simulink model "ackerman_modelo_parte1_neuronal"  (R2023b)
settings: Solver=FixedStepDiscrete  StartTime=0.0  StopTime=50  FixedStep=0.1  RelTol=1e-3
undefined symbols (not defined in the file or in its folder): Angular, Linear
libraries: neural x121, robotlib x15, fuzblock x1, robotcorelib x1
(part 4 of 5)

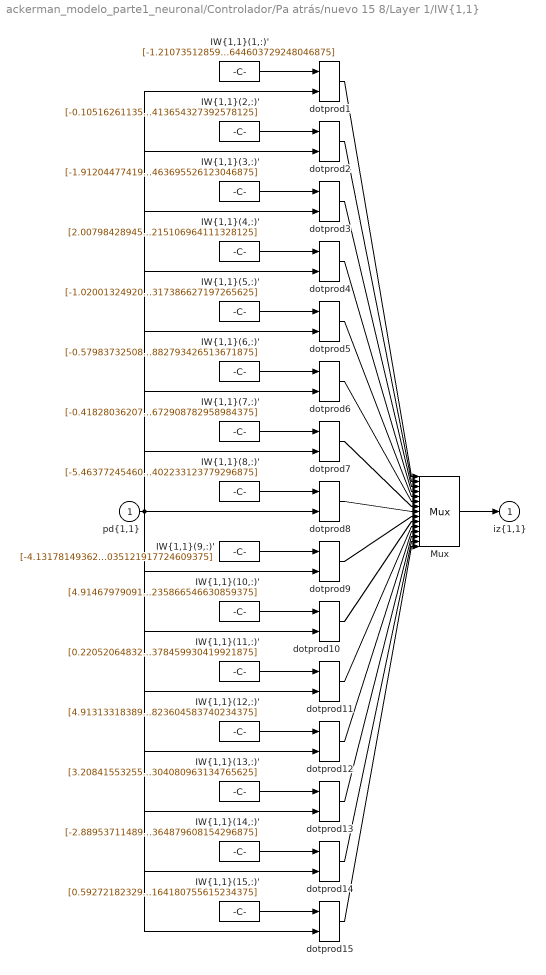
== system ackerman_modelo_parte1_neuronal/Controlador/Pa atrás/nuevo 15 8/Layer 1/IW{1,1} ==
  "pd{1,1}" : Inport  PortDimensions=12  SampleTime=0.1
      mask Display: e = 0.06;c1 = [120 230 180]/255;c2 = ([120 230 180]+0)/(256+128);c3 = ([120 230 180]+128)/(256+128);patch([0 1 1 0],[0 0 1 1],c1);patch([0 1 1 1-e 1-e 0+e],[0 0 1 1-e 0+e 0+e],c2);patch([0 0 1 1-e 0+e 0+e],[0 1 1 1-e 1-e 0+e],c3);plot([0 1 1 0 0],[0 0 1 1 0]);
  "IW{1,1}(1,:)'" : Constant  Value=[-1.2107351285968033227646856175852008163928985595703125;0.0982637498885013116467490590366651304066181182861328125;-0.5153760046711977071964838614803738892078399658203125;4.31122767760680147830498754046857357025146484375;3.85293074004639368723701409180648624897003173828125;-0.210691315343805418702771703465259633958339691162109375;2.04507854540902034301552703254856169223785400390625;-0.9143036407233731122090603093965910375118255615234375;-0.0603308152257395757800395585945807397365570068359375;-1.4964433902647422680587396826012991368770599365234375;0.70598829467948298610480151182855479419231414794921875;-3.888548718957604677370909485034644603729248046875]
      mask Display: e = 0.06;c1 = [120 150 230]/255;c2 = ([120 150 230]+0)/383;c3 = ([120 150 230]+128)/383;patch([0 1 1 0],[0 0 1 1],c1);patch([0 1 1 1-e 1-e 0+e],[0 0 1 1-e 0+e 0+e],c2);patch([0 0 1 1-e 0+e 0+e],[0 1 1 1-e 1-e 0+e],c3);plot([0 1 1 0 0],[0 0 1 1 0]);disp('Weights');
  "IW{1,1}(10,:)'" : Constant  Value=[4.91467979091452367157444314216263592243194580078125;4.34626894631366322840904103941284120082855224609375;2.404366244111241446290705425781197845935821533203125;-6.8842796230847458360813106992281973361968994140625;2.139509471626407588473739451728761196136474609375;3.83863946131409239370668728952296078205108642578125;-3.39886262811612649414882980636321008205413818359375;-3.524387185952170487013290767208673059940338134765625;3.065775570742113931288486128323711454868316650390625;1.4407812730284497160226919731940142810344696044921875;0.08745738485305031006955545080927549861371517181396484375;0.85647591674319922816493999562226235866546630859375]
      mask Display: e = 0.06;c1 = [120 150 230]/255;c2 = ([120 150 230]+0)/383;c3 = ([120 150 230]+128)/383;patch([0 1 1 0],[0 0 1 1],c1);patch([0 1 1 1-e 1-e 0+e],[0 0 1 1-e 0+e 0+e],c2);patch([0 0 1 1-e 0+e 0+e],[0 1 1 1-e 1-e 0+e],c3);plot([0 1 1 0 0],[0 0 1 1 0]);disp('Weights');
  "IW{1,1}(11,:)'" : Constant  Value=[0.2205206483206818557363249055924825370311737060546875;1.8123150518481307980067640528432093560695648193359375;0.7869633308428676254919764687656424939632415771484375;2.18414976750363099000651345704682171344757080078125;-3.05959657538790086306335069821216166019439697265625;2.11925190216866621284452776308171451091766357421875;-0.222273935716689352570796245345263741910457611083984375;-0.5932835817560018210059524790267460048198699951171875;0.9675585951395404560315682829241268336772918701171875;-2.879213642821424112838712972006760537624359130859375;-0.936850701180139910917432644055224955081939697265625;-0.99529495461161854308329566265456378459930419921875]
      mask Display: e = 0.06;c1 = [120 150 230]/255;c2 = ([120 150 230]+0)/383;c3 = ([120 150 230]+128)/383;patch([0 1 1 0],[0 0 1 1],c1);patch([0 1 1 1-e 1-e 0+e],[0 0 1 1-e 0+e 0+e],c2);patch([0 0 1 1-e 0+e 0+e],[0 1 1 1-e 1-e 0+e],c3);plot([0 1 1 0 0],[0 0 1 1 0]);disp('Weights');
  "IW{1,1}(12,:)'" : Constant  Value=[4.91313318389939457375703568686731159687042236328125;-0.2228704482321312851933470255971769802272319793701171875;1.48781041301915362140562137938104569911956787109375;2.11504413384102374351414255215786397457122802734375;-5.6137042363568081526636888156644999980926513671875;-0.868753373670580142373864873661659657955169677734375;3.59322897737675095442000383627600967884063720703125;0.54487347859706491970399611091124825179576873779296875;6.037217866595415927122303401120007038116455078125;-3.333595774710569781262847754987888038158416748046875;2.317143802646336236961133181466720998287200927734375;0.08013759538293162287825310841071768663823604583740234375]
      mask Display: e = 0.06;c1 = [120 150 230]/255;c2 = ([120 150 230]+0)/383;c3 = ([120 150 230]+128)/383;patch([0 1 1 0],[0 0 1 1],c1);patch([0 1 1 1-e 1-e 0+e],[0 0 1 1-e 0+e 0+e],c2);patch([0 0 1 1-e 0+e 0+e],[0 1 1 1-e 1-e 0+e],c3);plot([0 1 1 0 0],[0 0 1 1 0]);disp('Weights');
  "IW{1,1}(13,:)'" : Constant  Value=[3.2084155325522534241144967381842434406280517578125;4.08655173187908982157523496425710618495941162109375;-0.74005314094400909130655463741277344524860382080078125;-1.4115221687797758765015032622613944113254547119140625;-4.52962761692046544936829377547837793827056884765625;-3.25902700111771448376885018660686910152435302734375;-2.27197968931137861403612987487576901912689208984375;-1.6041119526664726624431978052598424255847930908203125;1.7664155094637392640066764215589500963687896728515625;-1.9371624002321834456807891911012120544910430908203125;4.80163975118690444787716842256486415863037109375;2.7784505359702027504908983246423304080963134765625]
      mask Display: e = 0.06;c1 = [120 150 230]/255;c2 = ([120 150 230]+0)/383;c3 = ([120 150 230]+128)/383;patch([0 1 1 0],[0 0 1 1],c1);patch([0 1 1 1-e 1-e 0+e],[0 0 1 1-e 0+e 0+e],c2);patch([0 0 1 1-e 0+e 0+e],[0 1 1 1-e 1-e 0+e],c3);plot([0 1 1 0 0],[0 0 1 1 0]);disp('Weights');
  "IW{1,1}(14,:)'" : Constant  Value=[-2.889537114898974135002163166063837707042694091796875;-1.048370824648822807745318641536869108676910400390625;-0.51568992051216977490213366763782687485218048095703125;0.0980394159708294632427083570291870273649692535400390625;0.1474327544041719451062277812525280751287937164306640625;-1.9644717917155867237255506552173756062984466552734375;-3.141171661324176245244643723708577454090118408203125;-2.1627338507038214032718315138481557369232177734375;-2.283212601949863529426920649711973965167999267578125;0.2879837913213993960681591488537378609180450439453125;-1.6861613409542035579846697146422229707241058349609375;-0.90119074943709509550870961902546696364879608154296875]
      mask Display: e = 0.06;c1 = [120 150 230]/255;c2 = ([120 150 230]+0)/383;c3 = ([120 150 230]+128)/383;patch([0 1 1 0],[0 0 1 1],c1);patch([0 1 1 1-e 1-e 0+e],[0 0 1 1-e 0+e 0+e],c2);patch([0 0 1 1-e 0+e 0+e],[0 1 1 1-e 1-e 0+e],c3);plot([0 1 1 0 0],[0 0 1 1 0]);disp('Weights');
  "IW{1,1}(15,:)'" : Constant  Value=[0.5927218232989857060744043337763287127017974853515625;6.05095360760331058003202997497282922267913818359375;5.70459075526748815576638662605546414852142333984375;1.0913370531196016077757349194143898785114288330078125;-6.16238780094926763553075943491421639919281005859375;3.14740655635683896917953461525030434131622314453125;1.6970071893540310536963033882784657180309295654296875;-1.74537787608898664615253437659703195095062255859375;0.214836119473990672101848531383438967168331146240234375;4.3552918607225450386977172456681728363037109375;3.99437144434348123667177787865512073040008544921875;3.0011419277898792046244125231169164180755615234375]
      mask Display: e = 0.06;c1 = [120 150 230]/255;c2 = ([120 150 230]+0)/383;c3 = ([120 150 230]+128)/383;patch([0 1 1 0],[0 0 1 1],c1);patch([0 1 1 1-e 1-e 0+e],[0 0 1 1-e 0+e 0+e],c2);patch([0 0 1 1-e 0+e 0+e],[0 1 1 1-e 1-e 0+e],c3);plot([0 1 1 0 0],[0 0 1 1 0]);disp('Weights');
  "IW{1,1}(2,:)'" : Constant  Value=[-0.1051626113599678780108348519206629134714603424072265625;-5.083606135239737255915315472520887851715087890625;2.00321524443686005412246231571771204471588134765625;0.86672090627960673980823003148543648421764373779296875;2.228908768658861117017977448995225131511688232421875;-0.80080397013559767582790982487495057284832000732421875;0.49174544290695099135746204410679638385772705078125;3.6915718186289350200013359426520764827728271484375;-1.19836535767401830554490516078658401966094970703125;-1.706882284913678216042853819089941680431365966796875;-0.822687260484902704860132871544919908046722412109375;0.70350327650940791546219088559155352413654327392578125]
      mask Display: e = 0.06;c1 = [120 150 230]/255;c2 = ([120 150 230]+0)/383;c3 = ([120 150 230]+128)/383;patch([0 1 1 0],[0 0 1 1],c1);patch([0 1 1 1-e 1-e 0+e],[0 0 1 1-e 0+e 0+e],c2);patch([0 0 1 1-e 0+e 0+e],[0 1 1 1-e 1-e 0+e],c3);plot([0 1 1 0 0],[0 0 1 1 0]);disp('Weights');
  "IW{1,1}(3,:)'" : Constant  Value=[-1.9120447741941515307217969166231341660022735595703125;-0.456778138788140608550492061112890951335430145263671875;0.61407563958637301215759407568839378654956817626953125;-0.59789275549836140566384301564539782702922821044921875;-3.52278262027996991179179531172849237918853759765625;2.111624613374857961645147952367551624774932861328125;-3.9493715623728125052593895816244184970855712890625;1.10848913770916279730727183050476014614105224609375;4.96544220863601548643373462255112826824188232421875;-2.521311409694160676764340678346343338489532470703125;-4.376974089342962059845376643352210521697998046875;2.135437127611392593706796105834655463695526123046875]
      mask Display: e = 0.06;c1 = [120 150 230]/255;c2 = ([120 150 230]+0)/383;c3 = ([120 150 230]+128)/383;patch([0 1 1 0],[0 0 1 1],c1);patch([0 1 1 1-e 1-e 0+e],[0 0 1 1-e 0+e 0+e],c2);patch([0 0 1 1-e 0+e 0+e],[0 1 1 1-e 1-e 0+e],c3);plot([0 1 1 0 0],[0 0 1 1 0]);disp('Weights');
  "IW{1,1}(4,:)'" : Constant  Value=[2.0079842894568162847690473427064716815948486328125;0.77019648946443652892668296772171743214130401611328125;3.1709271112167289885519494418986141681671142578125;-1.2126101810723934892877196034532971680164337158203125;-4.377744816317044040943073923699557781219482421875;3.143535997099470069571225394611246883869171142578125;6.37228009121002259007582324557006359100341796875;5.3420881020253947468745536752976477146148681640625;-0.1580693080755513069135531623032875359058380126953125;0.916039178029972145367310076835565268993377685546875;4.446636562875664111516016419045627117156982421875;0.85009214377447250843289339172770269215106964111328125]
      mask Display: e = 0.06;c1 = [120 150 230]/255;c2 = ([120 150 230]+0)/383;c3 = ([120 150 230]+128)/383;patch([0 1 1 0],[0 0 1 1],c1);patch([0 1 1 1-e 1-e 0+e],[0 0 1 1-e 0+e 0+e],c2);patch([0 0 1 1-e 0+e 0+e],[0 1 1 1-e 1-e 0+e],c3);plot([0 1 1 0 0],[0 0 1 1 0]);disp('Weights');
  "IW{1,1}(5,:)'" : Constant  Value=[-1.0200132492011257934194645713432691991329193115234375;2.115587292969216104410179468686692416667938232421875;0.058765464456745297727735533044324256479740142822265625;-0.9369911708232419034203530827653594315052032470703125;-0.8617614761682770296857825087499804794788360595703125;-2.436977052131390042433167764102108776569366455078125;-1.9178939983275438141419044768554158508777618408203125;-3.657381782514789403393251632223837077617645263671875;0.0727938413210702239819482883831369690597057342529296875;5.3628189763214226815080110100097954273223876953125;-1.9620170434064068132329339277930557727813720703125;0.60265908988629723896934820004389621317386627197265625]
      mask Display: e = 0.06;c1 = [120 150 230]/255;c2 = ([120 150 230]+0)/383;c3 = ([120 150 230]+128)/383;patch([0 1 1 0],[0 0 1 1],c1);patch([0 1 1 1-e 1-e 0+e],[0 0 1 1-e 0+e 0+e],c2);patch([0 0 1 1-e 0+e 0+e],[0 1 1 1-e 1-e 0+e],c3);plot([0 1 1 0 0],[0 0 1 1 0]);disp('Weights');
  "IW{1,1}(6,:)'" : Constant  Value=[-0.5798373250875332729492583894170820713043212890625;3.49037173488871221849194625974632799625396728515625;2.69385366427376293785300731542520225048065185546875;4.99342327369683491866680924431420862674713134765625;1.3203490130336168473235147757804952561855316162109375;0.68025931851506127312489979885867796838283538818359375;5.04882126855442958657249619136564433574676513671875;-2.352048108762541556160385880502872169017791748046875;-5.6367484957371818410365449381060898303985595703125;1.343725558897456817675220008823089301586151123046875;-1.028824242655661524992183331050910055637359619140625;-3.479813826287624589639335681567899882793426513671875]
      mask Display: e = 0.06;c1 = [120 150 230]/255;c2 = ([120 150 230]+0)/383;c3 = ([120 150 230]+128)/383;patch([0 1 1 0],[0 0 1 1],c1);patch([0 1 1 1-e 1-e 0+e],[0 0 1 1-e 0+e 0+e],c2);patch([0 0 1 1-e 0+e 0+e],[0 1 1 1-e 1-e 0+e],c3);plot([0 1 1 0 0],[0 0 1 1 0]);disp('Weights');
  "IW{1,1}(7,:)'" : Constant  Value=[-0.41828036207490260078856181280571036040782928466796875;-3.207646797774704960914959883666597306728363037109375;1.118927025324791824090198133490048348903656005859375;-0.85184466732525565557665458982228301465511322021484375;-0.507459282776808517922972896485589444637298583984375;-0.00546286069858389726483505199894352699629962444305419921875;-1.0917087277428538794055157268303446471691131591796875;1.6598742597553126643106224946677684783935546875;-2.34331138125278659600780883920378983020782470703125;-2.455131769084918591516952801612205803394317626953125;-1.2118189054765855505735316910431720316410064697265625;-2.27290972117965761611912967055104672908782958984375]
      mask Display: e = 0.06;c1 = [120 150 230]/255;c2 = ([120 150 230]+0)/383;c3 = ([120 150 230]+128)/383;patch([0 1 1 0],[0 0 1 1],c1);patch([0 1 1 1-e 1-e 0+e],[0 0 1 1-e 0+e 0+e],c2);patch([0 0 1 1-e 0+e 0+e],[0 1 1 1-e 1-e 0+e],c3);plot([0 1 1 0 0],[0 0 1 1 0]);disp('Weights');
  "IW{1,1}(8,:)'" : Constant  Value=[-5.46377245460134730592471896670758724212646484375;4.77850376478235272514893949846737086772918701171875;-3.063882030696078562215234342147596180438995361328125;1.7026186023976028760529288774705491960048675537109375;0.057268640450032416711056981739602633751928806304931640625;-3.043911938405681194552698798361234366893768310546875;-2.087085973080445189253850912791676819324493408203125;-0.6478883460483615408520563505589962005615234375;-1.6495490128681875585670013606431894004344940185546875;3.76449083714243304399360567913390696048736572265625;-2.061732774841388948772191724856384098529815673828125;0.440287490512660528718669183945166878402233123779296875]
      mask Display: e = 0.06;c1 = [120 150 230]/255;c2 = ([120 150 230]+0)/383;c3 = ([120 150 230]+128)/383;patch([0 1 1 0],[0 0 1 1],c1);patch([0 1 1 1-e 1-e 0+e],[0 0 1 1-e 0+e 0+e],c2);patch([0 0 1 1-e 0+e 0+e],[0 1 1 1-e 1-e 0+e],c3);plot([0 1 1 0 0],[0 0 1 1 0]);disp('Weights');
  "IW{1,1}(9,:)'" : Constant  Value=[-4.1317814936234071865328587591648101806640625;-0.54267309292749998927973820173065178096294403076171875;3.248198500675273603377490871935151517391204833984375;2.314857084656230856722913813428021967411041259765625;1.8523167152062758322728086568531580269336700439453125;1.9029771433222639753779503735131584107875823974609375;3.357464691081492258462048994260840117931365966796875;-1.8211175913287707128773718068259768187999725341796875;2.871623886888575949427604427910409867763519287109375;3.300857412961221815095314013888128101825714111328125;-8.9937746890157530543774555553682148456573486328125;2.118140016172025408280887859291397035121917724609375]
      mask Display: e = 0.06;c1 = [120 150 230]/255;c2 = ([120 150 230]+0)/383;c3 = ([120 150 230]+128)/383;patch([0 1 1 0],[0 0 1 1],c1);patch([0 1 1 1-e 1-e 0+e],[0 0 1 1-e 0+e 0+e],c2);patch([0 0 1 1-e 0+e 0+e],[0 1 1 1-e 1-e 0+e],c3);plot([0 1 1 0 0],[0 0 1 1 0]);disp('Weights');
  Mux : Mux  Inputs=15
      mask Display: e = 0.06;c1 = [120 150 230]/255;c2 = ([120 150 230]+0)/383;c3 = ([120 150 230]+128)/383;patch([0 1 1 0],[0 0 1 1],c1);patch([0 1 1 1-e 1-e 0+e],[0 0 1 1-e 0+e 0+e],c2);patch([0 0 1 1-e 0+e 0+e],[0 1 1 1-e 1-e 0+e],c3);plot([0 1 1 0 0],[0 0 1 1 0]);disp('Mux');
  dotprod{1..15} (15 alike) : neural/Weight Functions/dotprod
  "iz{1,1}" : Outport
      mask Display: e = 0.06;c1 = [120 230 180]/255;c2 = ([120 230 180]+0)/(256+128);c3 = ([120 230 180]+128)/(256+128);patch([0 1 1 0],[0 0 1 1],c1);patch([0 1 1 1-e 1-e 0+e],[0 0 1 1-e 0+e 0+e],c2);patch([0 0 1 1-e 0+e 0+e],[0 1 1 1-e 1-e 0+e],c3);plot([0 1 1 0 0],[0 0 1 1 0]);
  wires:
  Mux/1 -> "iz{1,1}"/1
  dotprod15/1 -> Mux/15
  "IW{1,1}(15,:)'"/1 -> dotprod15/1
  dotprod14/1 -> Mux/14
  "IW{1,1}(14,:)'"/1 -> dotprod14/1
  dotprod13/1 -> Mux/13
  "IW{1,1}(13,:)'"/1 -> dotprod13/1
  dotprod12/1 -> Mux/12
  "IW{1,1}(12,:)'"/1 -> dotprod12/1
  dotprod11/1 -> Mux/11
  "IW{1,1}(11,:)'"/1 -> dotprod11/1
  dotprod10/1 -> Mux/10
  "IW{1,1}(10,:)'"/1 -> dotprod10/1
  dotprod9/1 -> Mux/9
  "IW{1,1}(9,:)'"/1 -> dotprod9/1
  dotprod8/1 -> Mux/8
  "IW{1,1}(8,:)'"/1 -> dotprod8/1
  dotprod7/1 -> Mux/7
  "IW{1,1}(7,:)'"/1 -> dotprod7/1
  dotprod6/1 -> Mux/6
  "IW{1,1}(6,:)'"/1 -> dotprod6/1
  dotprod5/1 -> Mux/5
  "IW{1,1}(5,:)'"/1 -> dotprod5/1
  dotprod4/1 -> Mux/4
  "IW{1,1}(4,:)'"/1 -> dotprod4/1
  dotprod3/1 -> Mux/3
  "IW{1,1}(3,:)'"/1 -> dotprod3/1
  dotprod2/1 -> Mux/2
  "IW{1,1}(2,:)'"/1 -> dotprod2/1
  dotprod1/1 -> Mux/1
  "pd{1,1}"/1 -> dotprod15/2, dotprod14/2, dotprod13/2, dotprod12/2, dotprod11/2, dotprod10/2, dotprod9/2, dotprod8/2, dotprod7/2, dotprod6/2, dotprod5/2, dotprod4/2, dotprod3/2, dotprod2/2, dotprod1/2
  "IW{1,1}(1,:)'"/1 -> dotprod1/1

== system ackerman_modelo_parte1_neuronal/Controlador/Pa atrás/nuevo 15 8/Layer 2/Delays 1 ==
  "p{2}" : Inport  PortDimensions=15  SampleTime=0.1
      mask Display: e = 0.06;c1 = [120 230 180]/255;c2 = ([120 230 180]+0)/(256+128);c3 = ([120 230 180]+128)/(256+128);patch([0 1 1 0],[0 0 1 1],c1);patch([0 1 1 1-e 1-e 0+e],[0 0 1 1-e 0+e 0+e],c2);patch([0 0 1 1-e 0+e 0+e],[0 1 1 1-e 1-e 0+e],c3);plot([0 1 1 0 0],[0 0 1 1 0]);
  mux : Mux  Inputs=1
      mask Display: e = 0.06;c1 = [120 150 230]/255;c2 = ([120 150 230]+0)/383;c3 = ([120 150 230]+128)/383;patch([0 1 1 0],[0 0 1 1],c1);patch([0 1 1 1-e 1-e 0+e],[0 0 1 1-e 0+e 0+e],c2);patch([0 0 1 1-e 0+e 0+e],[0 1 1 1-e 1-e 0+e],c3);plot([0 1 1 0 0],[0 0 1 1 0]);disp('Mux')
  "pd{2,1}" : Outport
      mask Display: e = 0.06;c1 = [120 230 180]/255;c2 = ([120 230 180]+0)/(256+128);c3 = ([120 230 180]+128)/(256+128);patch([0 1 1 0],[0 0 1 1],c1);patch([0 1 1 1-e 1-e 0+e],[0 0 1 1-e 0+e 0+e],c2);patch([0 0 1 1-e 0+e 0+e],[0 1 1 1-e 1-e 0+e],c3);plot([0 1 1 0 0],[0 0 1 1 0]);
  wires:
  mux/1 -> "pd{2,1}"/1
  "p{2}"/1 -> mux/1

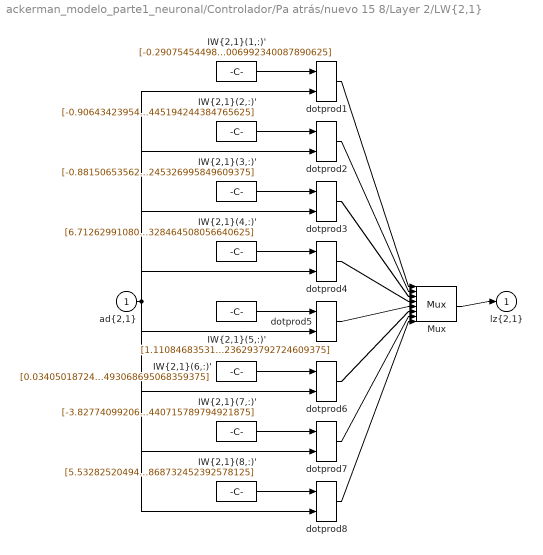
== system ackerman_modelo_parte1_neuronal/Controlador/Pa atrás/nuevo 15 8/Layer 2/LW{2,1} ==
  "ad{2,1}" : Inport  PortDimensions=15  SampleTime=0.1
      mask Display: e = 0.06;c1 = [120 230 180]/255;c2 = ([120 230 180]+0)/(256+128);c3 = ([120 230 180]+128)/(256+128);patch([0 1 1 0],[0 0 1 1],c1);patch([0 1 1 1-e 1-e 0+e],[0 0 1 1-e 0+e 0+e],c2);patch([0 0 1 1-e 0+e 0+e],[0 1 1 1-e 1-e 0+e],c3);plot([0 1 1 0 0],[0 0 1 1 0]);
  "IW{2,1}(1,:)'" : Constant  Value=[-0.29075454498602126829354119763593189418315887451171875;-0.98812314853822424964846504735760390758514404296875;0.711716360142102377750461528194136917591094970703125;0.90234703837315477503722149776876904070377349853515625;0.8126684356467970271609146948321722447872161865234375;-1.74164913561031564626091494574211537837982177734375;2.376338350655095243979531005606986582279205322265625;-0.92238662868760024071690395430778153240680694580078125;0.050248126972542821178091543288246612064540386199951171875;0.697568123453101041064883247599937021732330322265625;0.24326358760592459162808154360391199588775634765625;1.4125306528485872537004297555540688335895538330078125;0.539762979340757897972480350290425121784210205078125;2.241164585342918513788390555419027805328369140625;-0.96705426576078290512583635063492693006992340087890625]
      mask Display: e = 0.06;c1 = [120 150 230]/255;c2 = ([120 150 230]+0)/383;c3 = ([120 150 230]+128)/383;patch([0 1 1 0],[0 0 1 1],c1);patch([0 1 1 1-e 1-e 0+e],[0 0 1 1-e 0+e 0+e],c2);patch([0 0 1 1-e 0+e 0+e],[0 1 1 1-e 1-e 0+e],c3);plot([0 1 1 0 0],[0 0 1 1 0]);disp('weights');
  "IW{2,1}(2,:)'" : Constant  Value=[-0.906434239547387665680844293092377483844757080078125;-0.97475679697394335132543119470938108861446380615234375;-0.246538118535185868385184448925429023802280426025390625;-0.32752283539170956583319593846681527793407440185546875;-0.4956324478575202530095111796981655061244964599609375;-0.9529361012520130014280539398896507918834686279296875;0.8396212024492586412094397019245661795139312744140625;0.40149777369720640596284511047997511923313140869140625;4.930764217762515499998698942363262176513671875;0.19805403441289104460309999922174029052257537841796875;-0.38628534525447222325311713575501926243305206298828125;-0.2381274587910517659405940094075049273669719696044921875;-1.0404188470728821247490714085870422422885894775390625;-1.1803335311705318577679690861259587109088897705078125;-0.260692367339245001378600363750592805445194244384765625]
      mask Display: e = 0.06;c1 = [120 150 230]/255;c2 = ([120 150 230]+0)/383;c3 = ([120 150 230]+128)/383;patch([0 1 1 0],[0 0 1 1],c1);patch([0 1 1 1-e 1-e 0+e],[0 0 1 1-e 0+e 0+e],c2);patch([0 0 1 1-e 0+e 0+e],[0 1 1 1-e 1-e 0+e],c3);plot([0 1 1 0 0],[0 0 1 1 0]);disp('weights');
  "IW{2,1}(3,:)'" : Constant  Value=[-0.8815065356279401243000393151305615901947021484375;-2.172966928915788020759691789862699806690216064453125;0.6199742002492651948841739795170724391937255859375;1.59509701476742460357627351186238229274749755859375;-0.49622943112802442300335314939729869365692138671875;-0.52170933231938387830695091906818561255931854248046875;2.065467985535988315604072340647689998149871826171875;0.82253371757050819379486483740038238465785980224609375;-1.2643496444477679840900918861734680831432342529296875;-1.96010366548021419674796561594121158123016357421875;-5.18390017704719152646930524497292935848236083984375;1.799562773148688510360670989030040800571441650390625;-0.6347599582949925434149918146431446075439453125;3.202342757938753781132845688262023031711578369140625;2.29683725330840271539045716053806245326995849609375]
      mask Display: e = 0.06;c1 = [120 150 230]/255;c2 = ([120 150 230]+0)/383;c3 = ([120 150 230]+128)/383;patch([0 1 1 0],[0 0 1 1],c1);patch([0 1 1 1-e 1-e 0+e],[0 0 1 1-e 0+e 0+e],c2);patch([0 0 1 1-e 0+e 0+e],[0 1 1 1-e 1-e 0+e],c3);plot([0 1 1 0 0],[0 0 1 1 0]);disp('weights');
  "IW{2,1}(4,:)'" : Constant  Value=[6.712629910804526645051737432368099689483642578125;2.685481115080815772699907029164023697376251220703125;-5.22242244096624830262953764759004116058349609375;-4.64646258408361489955495926551520824432373046875;-7.8937720699343909558365339762531220912933349609375;-1.489316993595450444587413585395552217960357666015625;-0.0012315191105431166906925000148476101458072662353515625;-2.45356904701287703574053011834621429443359375;-4.3445683416797660214569987147115170955657958984375;9.4684540456393051499617286026477813720703125;-0.0495316660597107105701297768973745405673980712890625;7.388094109720238833460825844667851924896240234375;-7.59068304960720841023658067570067942142486572265625;-5.03963279409498188243787808460183441638946533203125;-5.151307660039666558304816135205328464508056640625]
      mask Display: e = 0.06;c1 = [120 150 230]/255;c2 = ([120 150 230]+0)/383;c3 = ([120 150 230]+128)/383;patch([0 1 1 0],[0 0 1 1],c1);patch([0 1 1 1-e 1-e 0+e],[0 0 1 1-e 0+e 0+e],c2);patch([0 0 1 1-e 0+e 0+e],[0 1 1 1-e 1-e 0+e],c3);plot([0 1 1 0 0],[0 0 1 1 0]);disp('weights');
  "IW{2,1}(5,:)'" : Constant  Value=[1.11084683531153505242627943516708910465240478515625;3.10043446301388403441023911000229418277740478515625;-1.0134746863376646874854714042157866060733795166015625;-1.770345289966909430035002515069209039211273193359375;-0.2142097084749770286027370502779376693069934844970703125;0.458936962485257449184672395858797244727611541748046875;-1.4054444424488057308053612359799444675445556640625;-0.68180700087420464949872211946058087050914764404296875;2.66641420630732550733910102280788123607635498046875;2.97762361888042192958891973830759525299072265625;3.51435835506861860011440512607805430889129638671875;-1.8125822622395599825750878153485246002674102783203125;1.022824479711518907976142145344056189060211181640625;-3.957830076097492710829328643740154802799224853515625;-2.850774159259832796209366279072128236293792724609375]
      mask Display: e = 0.06;c1 = [120 150 230]/255;c2 = ([120 150 230]+0)/383;c3 = ([120 150 230]+128)/383;patch([0 1 1 0],[0 0 1 1],c1);patch([0 1 1 1-e 1-e 0+e],[0 0 1 1-e 0+e 0+e],c2);patch([0 0 1 1-e 0+e 0+e],[0 1 1 1-e 1-e 0+e],c3);plot([0 1 1 0 0],[0 0 1 1 0]);disp('weights');
  "IW{2,1}(6,:)'" : Constant  Value=[0.0340501872422650786464970451561384834349155426025390625;-1.2045003328454597646413049005786888301372528076171875;-1.0884166133174826285312519758008420467376708984375;0.3230741253505637899934299639426171779632568359375;-0.69639101967878414001233977614901959896087646484375;-3.089062141086427626390786826959811151027679443359375;1.4201511556334318608918465542956255376338958740234375;-4.16687048502832357854686051723547279834747314453125;2.133040159648561751026818456011824309825897216796875;0.82352929019639253827023139820084907114505767822265625;-0.70289762206718087167445219165529124438762664794921875;-1.85767819933412869914945986238308250904083251953125;-7.98033056572949117679627306642942130565643310546875;-0.100894081643059629893599549177451990544795989990234375;-0.2212247530592440225571948531069210730493068695068359375]
      mask Display: e = 0.06;c1 = [120 150 230]/255;c2 = ([120 150 230]+0)/383;c3 = ([120 150 230]+128)/383;patch([0 1 1 0],[0 0 1 1],c1);patch([0 1 1 1-e 1-e 0+e],[0 0 1 1-e 0+e 0+e],c2);patch([0 0 1 1-e 0+e 0+e],[0 1 1 1-e 1-e 0+e],c3);plot([0 1 1 0 0],[0 0 1 1 0]);disp('weights');
  "IW{2,1}(7,:)'" : Constant  Value=[-3.827740992069419423415865821880288422107696533203125;-1.803984388809799721542503903037868440151214599609375;-1.822978187467001465194016418536193668842315673828125;5.97278661820225931222694271127693355083465576171875;-0.46747572108686774594588086984003894031047821044921875;2.19118725790278912057829074910841882228851318359375;5.15945985602581647100350892287679016590118408203125;-0.108402320187160394748815406273934058845043182373046875;4.174033651074037010175743489526212215423583984375;1.1081929070829825700883475292357616126537322998046875;-2.91075125748298457750706802471540868282318115234375;1.8023160883693958300710846742731519043445587158203125;0.30533085219115052577620872398256324231624603271484375;-5.911244402832952715698411338962614536285400390625;-1.1969564893468322974712236828054301440715789794921875]
      mask Display: e = 0.06;c1 = [120 150 230]/255;c2 = ([120 150 230]+0)/383;c3 = ([120 150 230]+128)/383;patch([0 1 1 0],[0 0 1 1],c1);patch([0 1 1 1-e 1-e 0+e],[0 0 1 1-e 0+e 0+e],c2);patch([0 0 1 1-e 0+e 0+e],[0 1 1 1-e 1-e 0+e],c3);plot([0 1 1 0 0],[0 0 1 1 0]);disp('weights');
  "IW{2,1}(8,:)'" : Constant  Value=[5.53282520494231189189804354100488126277923583984375;-2.37112003554331796095766549115069210529327392578125;4.7693327640777152254258908214978873729705810546875;-11.451800696300239224001416005194187164306640625;0.9340318427855525129643865511752665042877197265625;-0.368663405563989965418869587665540166199207305908203125;0.4524664595962504254345049048424698412418365478515625;-1.7536704038506008007658465430722571909427642822265625;-4.7963403600431373519086264423094689846038818359375;0.0099681725079447114357122927685850299894809722900390625;2.877485348191205272172510376549325883388519287109375;0.81593620475731665209195853094570338726043701171875;4.48453559542245283608963291044346988201141357421875;1.845719256720041556718570063821971416473388671875;3.259645459578770942954406564240343868732452392578125]
      mask Display: e = 0.06;c1 = [120 150 230]/255;c2 = ([120 150 230]+0)/383;c3 = ([120 150 230]+128)/383;patch([0 1 1 0],[0 0 1 1],c1);patch([0 1 1 1-e 1-e 0+e],[0 0 1 1-e 0+e 0+e],c2);patch([0 0 1 1-e 0+e 0+e],[0 1 1 1-e 1-e 0+e],c3);plot([0 1 1 0 0],[0 0 1 1 0]);disp('weights');
  Mux : Mux  Inputs=8
      mask Display: e = 0.06;c1 = [120 150 230]/255;c2 = ([120 150 230]+0)/383;c3 = ([120 150 230]+128)/383;patch([0 1 1 0],[0 0 1 1],c1);patch([0 1 1 1-e 1-e 0+e],[0 0 1 1-e 0+e 0+e],c2);patch([0 0 1 1-e 0+e 0+e],[0 1 1 1-e 1-e 0+e],c3);plot([0 1 1 0 0],[0 0 1 1 0]);disp('Mux');
  dotprod{1..8} (8 alike) : neural/Weight Functions/dotprod
  "lz{2,1}" : Outport
      mask Display: e = 0.06;c1 = [120 230 180]/255;c2 = ([120 230 180]+0)/(256+128);c3 = ([120 230 180]+128)/(256+128);patch([0 1 1 0],[0 0 1 1],c1);patch([0 1 1 1-e 1-e 0+e],[0 0 1 1-e 0+e 0+e],c2);patch([0 0 1 1-e 0+e 0+e],[0 1 1 1-e 1-e 0+e],c3);plot([0 1 1 0 0],[0 0 1 1 0]);
  wires:
  Mux/1 -> "lz{2,1}"/1
  dotprod8/1 -> Mux/8
  "IW{2,1}(8,:)'"/1 -> dotprod8/1
  dotprod7/1 -> Mux/7
  "IW{2,1}(7,:)'"/1 -> dotprod7/1
  dotprod6/1 -> Mux/6
  "IW{2,1}(6,:)'"/1 -> dotprod6/1
  dotprod5/1 -> Mux/5
  "IW{2,1}(5,:)'"/1 -> dotprod5/1
  dotprod4/1 -> Mux/4
  "IW{2,1}(4,:)'"/1 -> dotprod4/1
  dotprod3/1 -> Mux/3
  "IW{2,1}(3,:)'"/1 -> dotprod3/1
  dotprod2/1 -> Mux/2
  "IW{2,1}(2,:)'"/1 -> dotprod2/1
  dotprod1/1 -> Mux/1
  "ad{2,1}"/1 -> dotprod8/2, dotprod7/2, dotprod6/2, dotprod5/2, dotprod4/2, dotprod3/2, dotprod2/2, dotprod1/2
  "IW{2,1}(1,:)'"/1 -> dotprod1/1

== system ackerman_modelo_parte1_neuronal/Controlador/Pa atrás/nuevo 15 8/Layer 3/Delays 1 ==
  "p{3}" : Inport  PortDimensions=8  SampleTime=0.1
      mask Display: e = 0.06;c1 = [120 230 180]/255;c2 = ([120 230 180]+0)/(256+128);c3 = ([120 230 180]+128)/(256+128);patch([0 1 1 0],[0 0 1 1],c1);patch([0 1 1 1-e 1-e 0+e],[0 0 1 1-e 0+e 0+e],c2);patch([0 0 1 1-e 0+e 0+e],[0 1 1 1-e 1-e 0+e],c3);plot([0 1 1 0 0],[0 0 1 1 0]);
  mux : Mux  Inputs=1
      mask Display: e = 0.06;c1 = [120 150 230]/255;c2 = ([120 150 230]+0)/383;c3 = ([120 150 230]+128)/383;patch([0 1 1 0],[0 0 1 1],c1);patch([0 1 1 1-e 1-e 0+e],[0 0 1 1-e 0+e 0+e],c2);patch([0 0 1 1-e 0+e 0+e],[0 1 1 1-e 1-e 0+e],c3);plot([0 1 1 0 0],[0 0 1 1 0]);disp('Mux')
  "pd{3,2}" : Outport
      mask Display: e = 0.06;c1 = [120 230 180]/255;c2 = ([120 230 180]+0)/(256+128);c3 = ([120 230 180]+128)/(256+128);patch([0 1 1 0],[0 0 1 1],c1);patch([0 1 1 1-e 1-e 0+e],[0 0 1 1-e 0+e 0+e],c2);patch([0 0 1 1-e 0+e 0+e],[0 1 1 1-e 1-e 0+e],c3);plot([0 1 1 0 0],[0 0 1 1 0]);
  wires:
  mux/1 -> "pd{3,2}"/1
  "p{3}"/1 -> mux/1

== system ackerman_modelo_parte1_neuronal/Controlador/Pa atrás/nuevo 15 8/Layer 3/LW{3,2} ==
  "ad{3,2}" : Inport  PortDimensions=8  SampleTime=0.1
      mask Display: e = 0.06;c1 = [120 230 180]/255;c2 = ([120 230 180]+0)/(256+128);c3 = ([120 230 180]+128)/(256+128);patch([0 1 1 0],[0 0 1 1],c1);patch([0 1 1 1-e 1-e 0+e],[0 0 1 1-e 0+e 0+e],c2);patch([0 0 1 1-e 0+e 0+e],[0 1 1 1-e 1-e 0+e],c3);plot([0 1 1 0 0],[0 0 1 1 0]);
  "IW{3,2}(1,:)'" : Constant  Value=[-1.0331938380935119514703046661452390253543853759765625;0.209565686126775674313904573864419944584369659423828125;2.88807412630496340710806180140934884548187255859375;-0.88299286700145052098065434620366431772708892822265625;2.130932773028577198459743158309720456600189208984375;-0.372738243457286511084447511166217736899852752685546875;1.073500220734903365382706397213041782379150390625;1.0683849529528186561577740576467476785182952880859375]
      mask Display: e = 0.06;c1 = [120 150 230]/255;c2 = ([120 150 230]+0)/383;c3 = ([120 150 230]+128)/383;patch([0 1 1 0],[0 0 1 1],c1);patch([0 1 1 1-e 1-e 0+e],[0 0 1 1-e 0+e 0+e],c2);patch([0 0 1 1-e 0+e 0+e],[0 1 1 1-e 1-e 0+e],c3);plot([0 1 1 0 0],[0 0 1 1 0]);disp('weights');
  "IW{3,2}(2,:)'" : Constant  Value=[0.013546159522367949568089073864030069671571254730224609375;0.09338948559270195126646996186536853201687335968017578125;0.69941875664586550254142593985307030379772186279296875;0.308371856337186722729626353611820377409458160400390625;0.06363721643330506883007302576515940017998218536376953125;0.36216184455895683580450850058696232736110687255859375;-0.0836357800503415571569121311767958104610443115234375;-0.1742427424034324323631750530694262124598026275634765625]
      mask Display: e = 0.06;c1 = [120 150 230]/255;c2 = ([120 150 230]+0)/383;c3 = ([120 150 230]+128)/383;patch([0 1 1 0],[0 0 1 1],c1);patch([0 1 1 1-e 1-e 0+e],[0 0 1 1-e 0+e 0+e],c2);patch([0 0 1 1-e 0+e 0+e],[0 1 1 1-e 1-e 0+e],c3);plot([0 1 1 0 0],[0 0 1 1 0]);disp('weights');
  Mux : Mux  Inputs=2
      mask Display: e = 0.06;c1 = [120 150 230]/255;c2 = ([120 150 230]+0)/383;c3 = ([120 150 230]+128)/383;patch([0 1 1 0],[0 0 1 1],c1);patch([0 1 1 1-e 1-e 0+e],[0 0 1 1-e 0+e 0+e],c2);patch([0 0 1 1-e 0+e 0+e],[0 1 1 1-e 1-e 0+e],c3);plot([0 1 1 0 0],[0 0 1 1 0]);disp('Mux');
  dotprod1 : neural/Weight Functions/dotprod
  dotprod2 : neural/Weight Functions/dotprod
  "lz{3,2}" : Outport
      mask Display: e = 0.06;c1 = [120 230 180]/255;c2 = ([120 230 180]+0)/(256+128);c3 = ([120 230 180]+128)/(256+128);patch([0 1 1 0],[0 0 1 1],c1);patch([0 1 1 1-e 1-e 0+e],[0 0 1 1-e 0+e 0+e],c2);patch([0 0 1 1-e 0+e 0+e],[0 1 1 1-e 1-e 0+e],c3);plot([0 1 1 0 0],[0 0 1 1 0]);
  wires:
  Mux/1 -> "lz{3,2}"/1
  dotprod2/1 -> Mux/2
  "IW{3,2}(2,:)'"/1 -> dotprod2/1
  dotprod1/1 -> Mux/1
  "ad{3,2}"/1 -> dotprod2/2, dotprod1/2
  "IW{3,2}(1,:)'"/1 -> dotprod1/1

== system ackerman_modelo_parte1_neuronal/Controlador/Pa atrás/primer 15 8/Layer 1/Delays 1 ==
  "p{1}" : Inport  PortDimensions=12  SampleTime=0.1
      mask Display: e = 0.06;c1 = [120 230 180]/255;c2 = ([120 230 180]+0)/(256+128);c3 = ([120 230 180]+128)/(256+128);patch([0 1 1 0],[0 0 1 1],c1);patch([0 1 1 1-e 1-e 0+e],[0 0 1 1-e 0+e 0+e],c2);patch([0 0 1 1-e 0+e 0+e],[0 1 1 1-e 1-e 0+e],c3);plot([0 1 1 0 0],[0 0 1 1 0]);
  mux : Mux  Inputs=1
      mask Display: e = 0.06;c1 = [120 150 230]/255;c2 = ([120 150 230]+0)/383;c3 = ([120 150 230]+128)/383;patch([0 1 1 0],[0 0 1 1],c1);patch([0 1 1 1-e 1-e 0+e],[0 0 1 1-e 0+e 0+e],c2);patch([0 0 1 1-e 0+e 0+e],[0 1 1 1-e 1-e 0+e],c3);plot([0 1 1 0 0],[0 0 1 1 0]);disp('Mux')
  "pd{1,1}" : Outport
      mask Display: e = 0.06;c1 = [120 230 180]/255;c2 = ([120 230 180]+0)/(256+128);c3 = ([120 230 180]+128)/(256+128);patch([0 1 1 0],[0 0 1 1],c1);patch([0 1 1 1-e 1-e 0+e],[0 0 1 1-e 0+e 0+e],c2);patch([0 0 1 1-e 0+e 0+e],[0 1 1 1-e 1-e 0+e],c3);plot([0 1 1 0 0],[0 0 1 1 0]);
  wires:
  mux/1 -> "pd{1,1}"/1
  "p{1}"/1 -> mux/1
